simulink model "Quadrocopter_HIL_control"  (Simulink 7.4)
settings: Solver=ode45  StartTime=0.0  StopTime=7  RelTol=1e-3
values from neighbouring files (symbols this model uses):
  f1 = (I_y-I_z)/I_x    [quadrocopter_param.m]
  f2 = rot.J_z/I_x    [quadrocopter_param.m]
  f3 = (I_z-I_x)/I_y    [quadrocopter_param.m]
  f4 = rot.J_z/I_y    [quadrocopter_param.m]
  f5 = (I_x-I_y)/I_z    [quadrocopter_param.m]
  g = 9.81    [quadrocopter_param.m]
  I_x = elec.I_x+bat.I_x+2*boom.I_1x+2*boom.I_1y+2*mot.I_1x+2*mot.I_1y+                             2*rot.I_1x+2*rot.I_1y    [quadrocopter_param.m]
  I_y = elec.I_y+bat.I_y+2*boom.I_1x+2*boom.I_1y+2*mot.I_1x+2*mot.I_1y+                             2*rot.I_1x+2*rot.I_1y    [quadrocopter_param.m]
  I_z = elec.I_z+bat.I_z+4*boom.I_1z+4*mot.I_1z+4*rot.I_1z    [quadrocopter_param.m]
  m = m*1.2    [quadrocopter_param.m]
  phi0 = 0.15    [Quadrocopter_control_Driver.m]    (also in calc_stability.m = 0; control_two_angles_Driver.m; control_two_angles_and_yawrate_Driver.m; discrete_control_phi_theta_rpsi_Driver.m)
  r_phi0 = 0    [Quadrocopter_control_Driver.m]    (also in calc_stability.m; control_two_angles_Driver.m; control_two_angles_and_yawrate_Driver.m; discrete_control_phi_theta_rpsi_Driver.m)
  r_psi0 = 0    [Quadrocopter_control_Driver.m]    (also in calc_stability.m; control_two_angles_Driver.m = 0.01; control_two_angles_and_yawrate_Driver.m = 0.01; discrete_control_phi_theta_rpsi_Driver.m = 0.01)
  r_theta0 = 0    [Quadrocopter_control_Driver.m]    (also in calc_stability.m; control_two_angles_Driver.m; control_two_angles_and_yawrate_Driver.m; discrete_control_phi_theta_rpsi_Driver.m)
  theta0 = 0.15    [Quadrocopter_control_Driver.m]    (also in calc_stability.m = 0; control_two_angles_Driver.m; control_two_angles_and_yawrate_Driver.m; discrete_control_phi_theta_rpsi_Driver.m)
  Ts = 0.005    [quadrocopter_param.m]
undefined symbols (not defined in the file or in its folder): boom, Control_lib, HIL_Control
libraries: Copter_Library x6, simulink x3
settings Model: Creator=roczit00  LastModifiedBy=roczit00

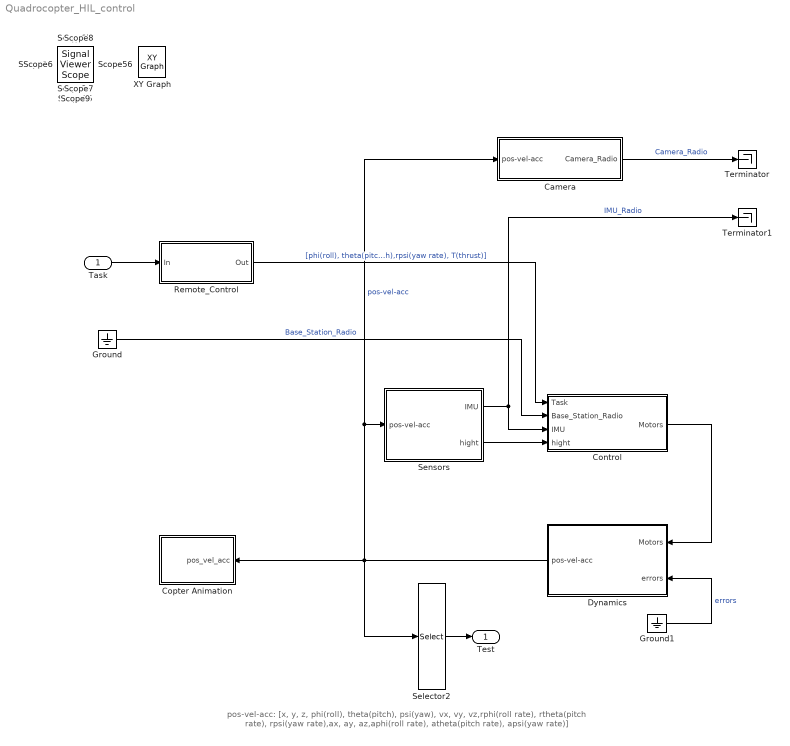
== system Quadrocopter_HIL_control ==
  note: pos-vel-acc: [x, y, z, phi(roll), theta(pitch), psi(yaw), vx, vy, vz,rphi(roll rate), rtheta(pitch rate), rpsi(yaw rate),ax, ay, az,aphi(roll rate), atheta(pitch rate), apsi(yaw rate)]
  Task : Inport  PortDimensions=4  OutDataType=fixdt(1, 16)  OutScaling=2^0
  Camera : Subsystem
  Control : Subsystem
  Copter Animation : Subsystem  mask(Quadrocopter Animation){AXES=[-100 100 -100 100 0 100], T_INT=1/25, K_VAR=Feste Position, K_POS=[5 0 1], K_ANGLE=27, A_ON=on, u_phi=on, u_theta=on, u_psi=on, u_x=off, u_y=off, u_z=off}
      mask prompts: AXES "Achsen Grenzen [xmin xmax ymin ymax zmin zmax]"; T_INT "Zeitintervall zwischen Aktualisierungen [s]:"; K_VAR "Kamera Art:"; K_POS "Ort der Kamera [xc yc zc]:"; K_ANGLE "Öffnungswinkel der Kamera [Grad]:"; A_ON "Animation Einschalten:"; u_phi "Use Input phi:"; u_theta "Use Input theta:"; u_psi "Use Input psi:"; u_x "Use Input x:"; u_y "Use Input y:"; u_z "Use Input z:"
      mask help: Erstellt eine 3-D animierte Ansicht eines Quadrocopters.
      mask init:
      | Config.axes = AXES;
      | Config.update = T_INT;
      | Config.camera_view = K_VAR;
      | Config.camera_pos = K_POS;
      | Config.view = K_ANGLE;
      | Config.Animenable = A_ON;
      | Config.phi = u_phi;
      | Config.theta = u_theta;
      | Config.psi = u_psi;
      | Config.x = u_x;
      | Config.y = u_y;
      | Config.z = u_z;
      mask Help:
      | <p>Dieser Block erstellt ein 3 dimensionales Fenster eines Quadrocopters.
      | 
      | <p><H4>Block Eingänge</H4>
      | Der Eingangsvektor bestehend aus:
      | <ul>
      | <li>X-Koordinate - Ort bezogen auf die X-Achse
      | <li>Y-Koordinate - Ort bezogen auf die Y-Achse
      | <li>Z-Koordinate - Ort bezogen auf die Z-Achse
      | <li>Psi - Yaw Drehung um die Z-Achse
      | <li>Phi - Roll Drehen um die Achse in Flugrichtung
      | <li>theta - pitch Neigung in Flugrichtung nach oben bzw. unten
      | </ul></p>
      mask StyleString: edit,edit,popup(Feste Position|Frei bewegbar),edit,edit,checkbox,checkbox,checkbox,checkbox,checkbox,checkbox,checkbox
  Dynamics : Subsystem
  Ground : Ground
  Ground1 : Ground
  Remote_Control : Subsystem
  Selector2 : Selector  InputPortWidth=19  IndexOptions=Index vector (dialog)  Indices=[4 5 6]  OutputSizes=1
  Sensors : Subsystem
  Terminator : Terminator
  Terminator1 : Terminator
  Test : Outport  OutDataType=fixdt(1, 16)  OutScaling=2^0
  Scope{,2,7..8,10,12} (6 alike) : SignalViewerScope  IOType=viewer  ZoomMode=yonly  RefreshTime=0.035000
      Scope settings: ShowLegends=on
      Scope10 settings: ShowLegends=on  SaveName=ScopeData10
      Scope12 settings: SaveName=ScopeData12
      Scope2 settings: ShowLegends=on  SaveName=ScopeData2
      Scope7 settings: SaveName=ScopeData7
      Scope8 settings: ShowLegends=on  SaveName=ScopeData8
  Scope1 : SignalViewerScope  IOType=viewer  ZoomMode=yonly  LegendLocations="1043.3333      702.66667             82      51.666667"  RefreshTime=0.035000
      settings: ShowLegends=on
  Scope11 : SignalViewerScope  IOType=viewer  ZoomMode=yonly  LegendLocations="260.3333           196            72      20.33333"  RefreshTime=0.103216
      settings: ShowLegends=on  YMin=-0.1  YMax=0.1  SaveName=ScopeData11
  Scope13 : SignalViewerScope  IOType=viewer  LegendLocations="990.2778      574.2778      159.6667      111.6667"  RefreshTime=0.035000
      settings: ShowLegends=on  SaveName=ScopeData13
  Scope14 : SignalViewerScope  IOType=viewer  ZoomMode=yonly  LegendLocations="242.3333           200            82      20.33333"  RefreshTime=0.148000
      settings: ShowLegends=on  YMin=-0.1  YMax=0.1  SaveName=ScopeData14
  Scope15 : SignalViewerScope  IOType=viewer  LegendLocations="233.3333           183            74      20.33333"  RefreshTime=0.035000
      settings: ShowLegends=on  SaveName=ScopeData15
  Scope16 : SignalViewerScope  IOType=viewer  LegendLocations="197.3333           136           106      67.33333"  RefreshTime=0.035000
      settings: ShowLegends=on  YMin=22  YMax=22  SaveName=ScopeData16
  Scope17 : SignalViewerScope  IOType=viewer  LegendLocations="180.3333           179           121      25.33333"  RefreshTime=0.035000
      settings: TickLabels=on  ShowDataMarkers=on  ShowLegends=on  TimeRange=0.01  SaveName=ScopeData17
  Scope3 : SignalViewerScope  IOType=viewer  LegendLocations="235.3333           136            72      67.33333"  RefreshTime=0.035000
      settings: ShowLegends=on  SaveName=ScopeData3
  Scope4 : SignalViewerScope  IOType=viewer  RefreshTime=0.035000
      settings: ShowLegends=on  SaveName=ScopeData4
  Scope5 : SignalViewerScope  IOType=viewer  LegendLocations="401.3333      415.6667           173      192.6667"  RefreshTime=0.035000
      settings: ShowLegends=on  SaveName=ScopeData5
  Scope6 : SignalViewerScope  IOType=viewer  RefreshTime=0.035000
      settings: ShowLegends=on  SaveName=ScopeData6
  Scope9 : SignalViewerScope  IOType=viewer  RefreshTime=0.035000
      settings: ShowLegends=on  SaveName=ScopeData9
  XY Graph : simulink/Sinks/XY Graph  IOType=viewer  SystemSampleTime=-1  xmin=-1  xmax=1  ymin=-1  ymax=1  st=-1
  wires:
  Sensors/1(IMU) -> Terminator1/1, Control/3(IMU)  "IMU_Radio"
  Sensors/2(hight) -> Control/4(hight)
  Ground1/1 -> Dynamics/2(errors)  "errors"
  Control/1(Motors) -> Dynamics/1(Motors)
  Dynamics/1(pos-vel-acc) -> Sensors/1(pos-vel-acc), Camera/1(pos-vel-acc), Selector2/1, Copter Animation/1(pos_vel_acc)  "pos-vel-acc"
  Camera/1(Camera_Radio) -> Terminator/1  "Camera_Radio"
  Ground/1 -> Control/2(Base_Station_Radio)  "Base_Station_Radio"
  Remote_Control/1(Out) -> Control/1(Task)  "[phi(roll), theta(pitch),rpsi(yaw rate), T(thrust)]"
  Selector2/1 -> Test/1
  Task/1 -> Remote_Control/1(In)

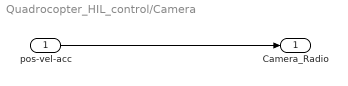
== system Quadrocopter_HIL_control/Camera ==
  pos-vel-acc : Inport  OutDataType=fixdt(1, 16)  OutScaling=2^0
  Camera_Radio : Outport  OutDataType=fixdt(1, 16)  OutScaling=2^0
  wires:
  pos-vel-acc/1 -> Camera_Radio/1

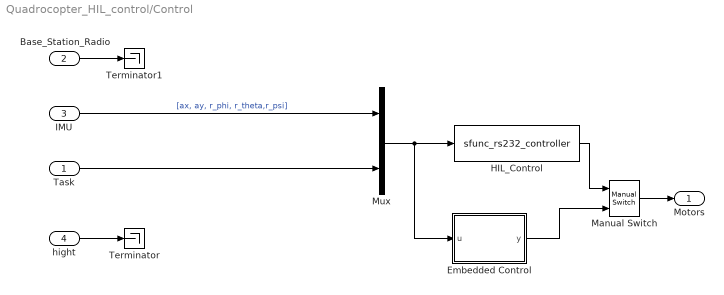
== system Quadrocopter_HIL_control/Control ==
  Task : Inport  PortDimensions=4  DataType=double  OutDataType=fixdt(1, 16)  OutScaling=2^0  OutDataTypeStr=double
  Base_Station_Radio : Inport  Port=2  OutDataType=fixdt(1, 16)  OutScaling=2^0
  IMU : Inport  Port=3  OutDataType=fixdt(1, 16)  OutScaling=2^0
  hight : Inport  Port=4  DataType=int16  OutDataType=fixdt(1, 16)  OutScaling=2^0  OutDataTypeStr=int16
  Embedded Control : Stateflow chart  AncestorBlock=Control_lib/Embedded Control
  HIL_Control : S-Function  AncestorBlock=Control_lib/HIL_Control  FunctionName=sfunc_rs232_controller  Parameters=Config  EnableBusSupport=off  mask{enabled=on}
      mask init:
      | Config.Enabled = enabled;
  Manual Switch : simulink/Signal Routing/Manual Switch  SystemSampleTime=-1  sw=1  action=0  varsize=off
  Mux : Mux  Inputs=2
  Terminator : Terminator
  Terminator1 : Terminator
  Motors : Outport  PortDimensions=4  OutDataType=fixdt(1, 16)  OutScaling=2^0
  wires:
  Base_Station_Radio/1 -> Terminator1/1
  hight/1 -> Terminator/1
  Mux/1 -> HIL_Control/1, Embedded Control/1(u)
  IMU/1 -> Mux/1  "[ax, ay, r_phi, r_theta,r_psi]"
  HIL_Control/1 -> Manual Switch/1
  Manual Switch/1 -> Motors/1
  Embedded Control/1(y) -> Manual Switch/2
  Task/1 -> Mux/2

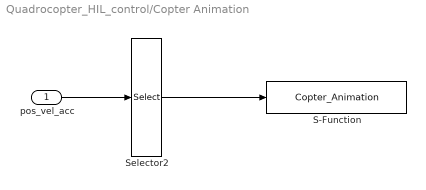
== system Quadrocopter_HIL_control/Copter Animation ==
  pos_vel_acc : Inport  PortDimensions=19  OutDataType=sfix(16)  OutScaling=2^0
  S-Function : S-Function  FunctionName=Copter_Animation  Parameters=Config  EnableBusSupport=off
  Selector2 : Selector  InputPortWidth=19  IndexOptions=Index vector (dialog)  Indices=[1 2 3 4 5 6]  OutputSizes=1
  wires:
  pos_vel_acc/1 -> Selector2/1
  Selector2/1 -> S-Function/1

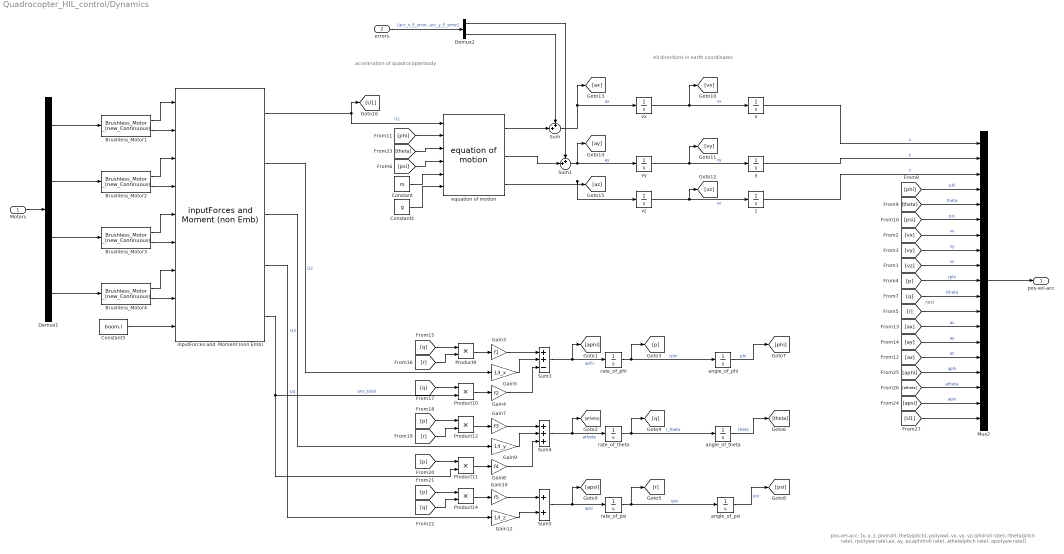
== system Quadrocopter_HIL_control/Dynamics ==
  note: rpsi
  note: pos-vel-acc: [x, y, z, phi(roll), theta(pitch), psi(yaw), vx, vy, vz,rphi(roll rate), rtheta(pitch rate), rpsi(yaw rate),ax, ay, az,aphi(roll rate), atheta(pitch rate), apsi(yaw rate)]
  note: All directions in earth coordinates
  note: acceleration of quadrocopterbody
  Motors : Inport  OutDataType=fixdt(1, 16)  OutScaling=2^0
  errors : Inport  Port=2  OutDataType=fixdt(1, 16)  OutScaling=2^0
  Brushless_Motor1 : Copter_Library/Brushless_Motor _(new_Continuous)  SystemSampleTime=-1  M_error=1
  Brushless_Motor2 : Copter_Library/Brushless_Motor _(new_Continuous)  SystemSampleTime=-1  M_error=1.03
  Brushless_Motor3 : Copter_Library/Brushless_Motor _(new_Continuous)  SystemSampleTime=-1  M_error=1
  Brushless_Motor4 : Copter_Library/Brushless_Motor _(new_Continuous)  SystemSampleTime=-1  M_error=1
  Constant : Constant  Value=m  OutDataType=fixdt(1, 16)  OutScaling=2^0
  Constant1 : Constant  Value=g  OutDataType=fixdt(1, 16)  OutScaling=2^0
  Constant3 : Constant  Value=boom.l  OutDataType=fixdt(1, 16)  OutScaling=2^0
  Demux1 : Demux
  Demux2 : Demux  Outputs=2
  Gain10 : Gain  Gain=f5  ParameterDataType=fixdt(1, 16)  ParameterScaling=2^0  OutDataType=fixdt(1, 16)  OutScaling=2^0
  Gain12 : Gain  Gain=1/I_z  ParameterDataType=fixdt(1, 16)  ParameterScaling=2^0  OutDataType=fixdt(1, 16)  OutScaling=2^0
  Gain3 : Gain  Gain=f1  ParameterDataType=fixdt(1, 16)  ParameterScaling=2^0  OutDataType=fixdt(1, 16)  OutScaling=2^0
  Gain4 : Gain  Gain=f2  ParameterDataType=fixdt(1, 16)  ParameterScaling=2^0  OutDataType=fixdt(1, 16)  OutScaling=2^0
  Gain5 : Gain  Gain=1/I_x  ParameterDataType=fixdt(1, 16)  ParameterScaling=2^0  OutDataType=fixdt(1, 16)  OutScaling=2^0
  Gain7 : Gain  Gain=f3  ParameterDataType=fixdt(1, 16)  ParameterScaling=2^0  OutDataType=fixdt(1, 16)  OutScaling=2^0
  Gain8 : Gain  Gain=f4  ParameterDataType=fixdt(1, 16)  ParameterScaling=2^0  OutDataType=fixdt(1, 16)  OutScaling=2^0
  Gain9 : Gain  Gain=1/I_y  ParameterDataType=fixdt(1, 16)  ParameterScaling=2^0  OutDataType=fixdt(1, 16)  OutScaling=2^0
  Mux2 : Mux  Inputs=19
  Product{9..12,14} (5 alike) : Product  OutDataType=fixdt(1, 16)  OutScaling=2^0  RndMeth=Zero
  Sum : Sum  Inputs=++|  OutDataType=fixdt(1, 16)  OutScaling=2^0
  Sum1 : Sum  Inputs=++|  OutDataType=fixdt(1, 16)  OutScaling=2^0
  Sum3 : Sum  Inputs=++-  OutDataType=fixdt(1, 16)  OutScaling=2^0
  Sum4 : Sum  Inputs=+++  OutDataType=fixdt(1, 16)  OutScaling=2^0
  Sum5 : Sum  OutDataType=fixdt(1, 16)  OutScaling=2^0
  angle_of_phi : Integrator  InitialCondition=phi0
  angle_of_psi : Integrator
  angle_of_theta : Integrator  InitialCondition=theta0
  equation of motion : Copter_Library/equation of motion  SystemSampleTime=-1
  inputForces and  Moment (non Emb) : Copter_Library/inputForces and  Moment (non Emb)  SystemSampleTime=-1
  rate_of_phi : Integrator  InitialCondition=r_phi0
  rate_of_psi : Integrator  InitialCondition=r_psi0
  rate_of_theta : Integrator  InitialCondition=r_theta0
  vx : Integrator
  vy : Integrator
  vz : Integrator
  x : Integrator
  y : Integrator
  z : Integrator
  pos-vel-acc : Outport  OutDataType=fixdt(1, 16)  OutScaling=2^0
  wires:
  [apsi] -> Mux2/18  "apsi"
  [atheta] -> Mux2/17  "atheta"
  [aphi] -> Mux2/16  "aphi"
  [az] -> Mux2/15  "az"
  [ay] -> Mux2/14  "ay"
  [ax] -> Mux2/13  "ax"
  [r] -> Mux2/12
  [q] -> Mux2/11  "rtheta"
  [p] -> Mux2/10  "rphi"
  [vz] -> Mux2/9  "vz"
  [vy] -> Mux2/8  "vy"
  [vx] -> Mux2/7  "vx"
  [psi] -> Mux2/6  "psi"
  [theta] -> Mux2/5  "theta"
  [phi] -> Mux2/4  "phi"
  z/1 -> Mux2/3  "z"
  Mux2/1 -> pos-vel-acc/1
  errors/1 -> Demux2/1  "[acc_x_E_error, acc_y_E_error]"
  Motors/1 -> Demux1/1
  Demux1/3 -> Brushless_Motor3/1
  Demux1/4 -> Brushless_Motor4/1
  Demux1/2 -> Brushless_Motor2/1
  Demux1/1 -> Brushless_Motor1/1
  vx/1 -> [vx], x/1  "vx"
  vy/1 -> [vy], y/1  "vy"
  vz/1 -> [vz], z/1  "vz"
  Constant3/1 -> inputForces and  Moment (non Emb)/9
  Sum5/1 -> [apsi], rate_of_psi/1  "apsi"
  inputForces and  Moment (non Emb)/4 -> Gain12/1  "U4"
  Gain12/1 -> Sum5/2
  Gain10/1 -> Sum5/1
  Product14/1 -> Gain10/1
  [q] -> Product14/2
  [p] -> Product14/1
  Sum4/1 -> [atheta], rate_of_theta/1  "atheta"
  inputForces and  Moment (non Emb)/3 -> Gain9/1  "U3"
  Gain8/1 -> Sum4/3
  Gain9/1 -> Sum4/2
  Product11/1 -> Gain8/1
  [p] -> Product11/1
  Gain7/1 -> Sum4/1
  Product12/1 -> Gain7/1
  [r] -> Product12/2
  [p] -> Product12/1
  Sum3/1 -> [aphi], rate_of_phi/1  "aphi"
  Gain4/1 -> Sum3/3
  Gain5/1 -> Sum3/2
  inputForces and  Moment (non Emb)/2 -> Gain5/1  "U2"
  Product10/1 -> Gain4/1
  [q] -> Product10/1
  Gain3/1 -> Sum3/1
  Product9/1 -> Gain3/1
  [r] -> Product9/2
  [q] -> Product9/1
  inputForces and  Moment (non Emb)/5 -> Product11/2, Product10/2  "anv_total"
  angle_of_phi/1 -> [phi]  "phi"
  angle_of_theta/1 -> [theta]  "theta"
  angle_of_psi/1 -> [psi]  "psi"
  rate_of_phi/1 -> [p], angle_of_phi/1  "rphi"
  rate_of_theta/1 -> angle_of_theta/1, [q]  "r_theta"
  rate_of_psi/1 -> angle_of_psi/1, [r]  "rpsi"
  Brushless_Motor1/1 -> inputForces and  Moment (non Emb)/1
  Brushless_Motor1/2 -> inputForces and  Moment (non Emb)/2
  Brushless_Motor2/1 -> inputForces and  Moment (non Emb)/3
  Brushless_Motor2/2 -> inputForces and  Moment (non Emb)/4
  Brushless_Motor3/1 -> inputForces and  Moment (non Emb)/5
  Brushless_Motor3/2 -> inputForces and  Moment (non Emb)/6
  Brushless_Motor4/1 -> inputForces and  Moment (non Emb)/7
  Brushless_Motor4/2 -> inputForces and  Moment (non Emb)/8
  x/1 -> Mux2/1  "x"
  y/1 -> Mux2/2  "y"
  Sum1/1 -> [ay], vy/1  "ay"
  Sum/1 -> [ax], vx/1  "ax"
  Demux2/2 -> Sum/1
  Demux2/1 -> Sum1/1
  equation of motion/3 -> [az], vz/1
  equation of motion/2 -> Sum1/2
  equation of motion/1 -> Sum/2
  inputForces and  Moment (non Emb)/1 -> equation of motion/1, [U1]  "U1"
  [phi] -> equation of motion/2
  [theta] -> equation of motion/3
  [psi] -> equation of motion/4
  Constant/1 -> equation of motion/5
  Constant1/1 -> equation of motion/6
  [U1] -> Mux2/19

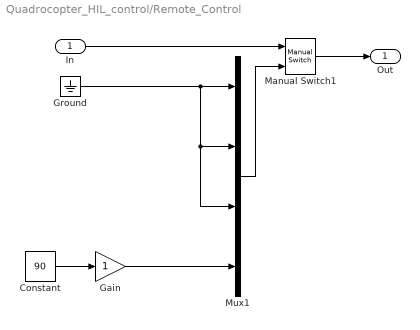
== system Quadrocopter_HIL_control/Remote_Control ==
  In : Inport  OutDataType=fixdt(1, 16)  OutScaling=2^0
  Constant : Constant  Value=90  OutDataType=fixdt(1, 16)  OutScaling=2^0
  Gain : Gain  ParameterDataType=fixdt(1, 16)  ParameterScaling=2^0  OutDataType=fixdt(1, 16)  OutScaling=2^0
  Ground : Ground
  Manual Switch1 : simulink/Signal Routing/Manual Switch  SystemSampleTime=-1  sw=0  action=0  varsize=off
  Mux1 : Mux
  Out : Outport  OutDataType=fixdt(1, 16)  OutScaling=2^0
  wires:
  In/1 -> Manual Switch1/1
  Mux1/1 -> Manual Switch1/2
  Ground/1 -> Mux1/1, Mux1/2, Mux1/3
  Manual Switch1/1 -> Out/1
  Gain/1 -> Mux1/4
  Constant/1 -> Gain/1

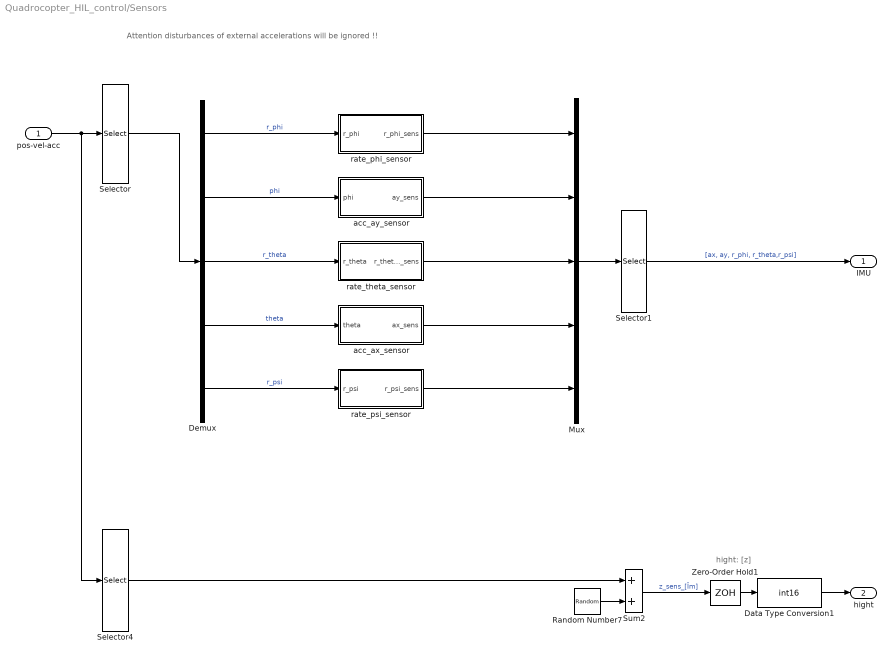
== system Quadrocopter_HIL_control/Sensors ==
  note: hight: [z]
  note: Attention disturbances of external accelerations will be ignored !!
  pos-vel-acc : Inport  PortDimensions=19  OutDataType=fixdt(1, 16)  OutScaling=2^0
  Data Type Conversion1 : DataTypeConversion  OutDataTypeMode=int16  OutDataType=fixdt(1, 16)  OutScaling=2^0  OutDataTypeStr=int16  RndMeth=Round
  Demux : Demux  Outputs=5
  Mux : Mux  Inputs=5
  Random Number7 : RandomNumber  Variance=0  SampleTime=Ts
  Selector : Selector  InputPortWidth=19  IndexOptions=Index vector (dialog)  Indices=[10 4 11 5 12]  OutputSizes=1
  Selector1 : Selector  InputPortWidth=5  IndexOptions=Index vector (dialog)  Indices=[4 2 1 3 5]  OutputSizes=1
  Selector4 : Selector  InputPortWidth=19  IndexOptions=Index vector (dialog)  Indices=[3]  OutputSizes=1
  Sum2 : Sum  OutDataType=fixdt(1, 16)  OutScaling=2^0
  Zero-Order Hold1 : ZeroOrderHold  SampleTime=Ts
  acc_ax_sensor : Subsystem
  acc_ay_sensor : Subsystem
  rate_phi_sensor : Subsystem
  rate_psi_sensor : Subsystem
  rate_theta_sensor : Subsystem
  IMU : Outport  OutDataType=fixdt(1, 16)  OutScaling=2^0
  hight : Outport  Port=2  OutDataType=fixdt(1, 16)  OutScaling=2^0
  wires:
  Random Number7/1 -> Sum2/2
  pos-vel-acc/1 -> Selector/1, Selector4/1
  Selector/1 -> Demux/1
  Selector4/1 -> Sum2/1
  Sum2/1 -> Zero-Order Hold1/1  "z_sens_[Ïm]"
  Zero-Order Hold1/1 -> Data Type Conversion1/1
  Data Type Conversion1/1 -> hight/1
  rate_phi_sensor/1(r_phi_sens) -> Mux/1
  acc_ay_sensor/1(ay_sens) -> Mux/2
  rate_theta_sensor/1(r_theta_sens) -> Mux/3
  acc_ax_sensor/1(ax_sens) -> Mux/4
  rate_psi_sensor/1(r_psi_sens) -> Mux/5
  Demux/1 -> rate_phi_sensor/1(r_phi)  "r_phi"
  Demux/2 -> acc_ay_sensor/1(phi)  "phi"
  Demux/3 -> rate_theta_sensor/1(r_theta)  "r_theta"
  Demux/4 -> acc_ax_sensor/1(theta)  "theta"
  Demux/5 -> rate_psi_sensor/1(r_psi)  "r_psi"
  Mux/1 -> Selector1/1
  Selector1/1 -> IMU/1  "[ax, ay, r_phi, r_theta,r_psi]"

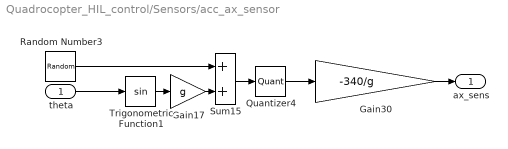
== system Quadrocopter_HIL_control/Sensors/acc_ax_sensor ==
  theta : Inport  OutDataType=fixdt(1, 16)  OutScaling=2^0
  Gain17 : Gain  Gain=g  ParameterDataType=fixdt(1, 16)  ParameterScaling=2^0  OutDataType=fixdt(1, 16)  OutScaling=2^0
  Gain30 : Gain  Gain=-340/g  ParameterDataType=fixdt(1, 16)  ParameterScaling=2^0  OutDataType=fixdt(1, 16)  OutScaling=2^0
  Quantizer4 : Quantizer  QuantizationInterval=g/340  SampleTime=Ts
  Random Number3 : RandomNumber  Variance=0.0003  Seed=676  SampleTime=Ts
  Sum15 : Sum  OutDataType=fixdt(1, 16)  OutScaling=2^0
  Trigonometric Function1 : Trigonometry
  ax_sens : Outport  OutDataType=fixdt(1, 16)  OutScaling=2^0
  wires:
  Random Number3/1 -> Sum15/1
  Sum15/1 -> Quantizer4/1
  Trigonometric Function1/1 -> Gain17/1
  Gain17/1 -> Sum15/2
  Quantizer4/1 -> Gain30/1
  theta/1 -> Trigonometric Function1/1
  Gain30/1 -> ax_sens/1

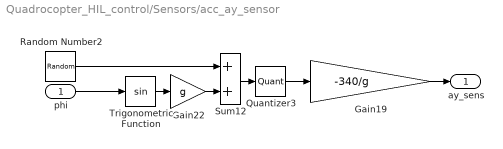
== system Quadrocopter_HIL_control/Sensors/acc_ay_sensor ==
  phi : Inport  OutDataType=fixdt(1, 16)  OutScaling=2^0
  Gain19 : Gain  Gain=-340/g  ParameterDataType=fixdt(1, 16)  ParameterScaling=2^0  OutDataType=fixdt(1, 16)  OutScaling=2^0
  Gain22 : Gain  Gain=g  ParameterDataType=fixdt(1, 16)  ParameterScaling=2^0  OutDataType=fixdt(1, 16)  OutScaling=2^0
  Quantizer3 : Quantizer  QuantizationInterval=g/340  SampleTime=Ts
  Random Number2 : RandomNumber  Variance=0.0003  Seed=4564  SampleTime=0.01
  Sum12 : Sum  OutDataType=fixdt(1, 16)  OutScaling=2^0
  Trigonometric Function : Trigonometry
  ay_sens : Outport  OutDataType=fixdt(1, 16)  OutScaling=2^0
  wires:
  Random Number2/1 -> Sum12/1
  Sum12/1 -> Quantizer3/1
  Trigonometric Function/1 -> Gain22/1
  Gain22/1 -> Sum12/2
  Quantizer3/1 -> Gain19/1
  phi/1 -> Trigonometric Function/1
  Gain19/1 -> ay_sens/1

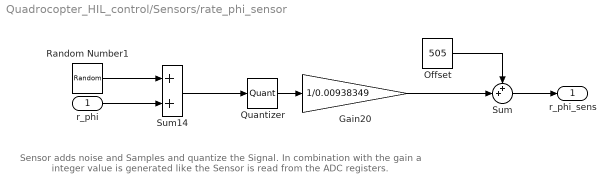
== system Quadrocopter_HIL_control/Sensors/rate_phi_sensor ==
  note: Sensor adds noise and Samples and quantize the Signal. In combination with the gain a integer value is generated
      | like the Sensor is read from the ADC registers.
  r_phi : Inport  OutDataType=fixdt(1, 16)  OutScaling=2^0
  Gain20 : Gain  Gain=1/0.00938349  ParameterDataType=fixdt(1, 16)  ParameterScaling=2^0  OutDataType=fixdt(1, 16)  OutScaling=2^0
  Offset : Constant  Value=505  OutDataType=fixdt(1, 16)  OutScaling=2^0
  Quantizer : Quantizer  QuantizationInterval=0.00938349  SampleTime=Ts
  Random Number1 : RandomNumber  Variance=3.0462e-8  Seed=45632  SampleTime=0.01
  Sum : Sum  Inputs=++|  OutDataType=fixdt(1, 16)  OutScaling=2^0
  Sum14 : Sum  OutDataType=fixdt(1, 16)  OutScaling=2^0
  r_phi_sens : Outport  OutDataType=fixdt(1, 16)  OutScaling=2^0
  wires:
  Random Number1/1 -> Sum14/1
  Sum14/1 -> Quantizer/1
  Quantizer/1 -> Gain20/1
  r_phi/1 -> Sum14/2
  Gain20/1 -> Sum/2
  Offset/1 -> Sum/1
  Sum/1 -> r_phi_sens/1

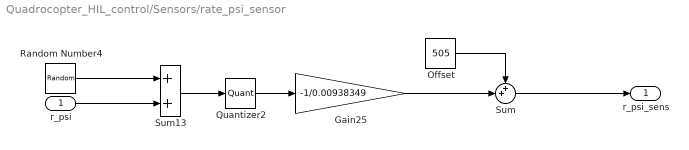
== system Quadrocopter_HIL_control/Sensors/rate_psi_sensor ==
  r_psi : Inport  OutDataType=fixdt(1, 16)  OutScaling=2^0
  Gain25 : Gain  Gain=-1/0.00938349  ParameterDataType=fixdt(1, 16)  ParameterScaling=2^0  OutDataType=fixdt(1, 16)  OutScaling=2^0
  Offset : Constant  Value=505  OutDataType=fixdt(1, 16)  OutScaling=2^0
  Quantizer2 : Quantizer  QuantizationInterval=0.00938349  SampleTime=Ts
  Random Number4 : RandomNumber  Variance=3.0462e-8  Seed=1634  SampleTime=0.01
  Sum : Sum  Inputs=++|  OutDataType=fixdt(1, 16)  OutScaling=2^0
  Sum13 : Sum  OutDataType=fixdt(1, 16)  OutScaling=2^0
  r_psi_sens : Outport  OutDataType=fixdt(1, 16)  OutScaling=2^0
  wires:
  Random Number4/1 -> Sum13/1
  Sum13/1 -> Quantizer2/1
  Quantizer2/1 -> Gain25/1
  r_psi/1 -> Sum13/2
  Offset/1 -> Sum/1
  Gain25/1 -> Sum/2
  Sum/1 -> r_psi_sens/1

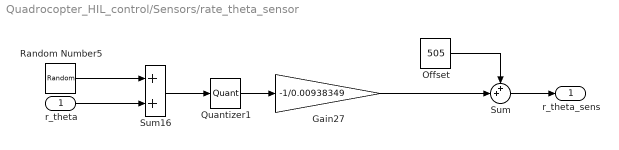
== system Quadrocopter_HIL_control/Sensors/rate_theta_sensor ==
  r_theta : Inport  OutDataType=fixdt(1, 16)  OutScaling=2^0
  Gain27 : Gain  Gain=-1/0.00938349  ParameterDataType=fixdt(1, 16)  ParameterScaling=2^0  OutDataType=fixdt(1, 16)  OutScaling=2^0
  Offset : Constant  Value=505  OutDataType=fixdt(1, 16)  OutScaling=2^0
  Quantizer1 : Quantizer  QuantizationInterval=0.00938349  SampleTime=Ts
  Random Number5 : RandomNumber  Variance=3.0462e-8  Seed=4731  SampleTime=0.01
  Sum : Sum  Inputs=++|  OutDataType=fixdt(1, 16)  OutScaling=2^0
  Sum16 : Sum  OutDataType=fixdt(1, 16)  OutScaling=2^0
  r_theta_sens : Outport  OutDataType=fixdt(1, 16)  OutScaling=2^0
  wires:
  Random Number5/1 -> Sum16/1
  Sum16/1 -> Quantizer1/1
  Quantizer1/1 -> Gain27/1
  r_theta/1 -> Sum16/2
  Offset/1 -> Sum/1
  Gain27/1 -> Sum/2
  Sum/1 -> r_theta_sens/1

== matlab function Control/Embedded Control ==
  data: u input double; y output double
function y = fcn(u)
%#eml
persistent phi_filt theta_filt M1 M2 M3 M4
%  first time initialization
if isempty(M1) 
    M1=int8(0);
end
if isempty(M2) 
    M2=int8(0);
end
if isempty(M3) 
    M3=int8(0);
end
if isempty(M4) 
    M4=int8(0);
end
if isempty(phi_filt) 
    phi_filt=0.15;
end
if isempty(theta_filt) 
    theta_filt=0.15;
end
Ts = 0.01;
Gyro_offset = 505;
% copy inputs to variables with easy to know names
Gyro_phi =  u(3)-Gyro_offset;
acc_ay = u(2);
Gyro_theta = u(4)-Gyro_offset;
acc_ax = u(1);
Gyro_psi = u(5)-Gyro_offset;
thrust = u(9);
theta_set = u(7);
phi_set = u(6);
r_psi_set = u(8);

% Set outputs to Values calculated last sample time
y = double([M1;M2;M3;M4]);

% Convert setpoint values to angles and rates
%(int16)(maxPitchAngle*(int32)(copterState->remotePitchRaw-128)/maxRemotePitch);
% Filter berechnen - ! deaktivated
phi_filt = acc_ay * 0.028852941 / 9.81; %phi_filt +Ts*((Gyro_phi * 0.00938349) + (acc_ay * 0.028852941 / 9.81 - phi_filt)*10);
theta_filt = acc_ax * 0.028852941 / 9.81;%theta_filt +Ts*((Gyro_theta * 0.00938349) + (acc_ax * 0.028852941 / 9.81 - theta_filt)*10);
% e-phi
e_phi=-(Gyro_phi * 0.00938349)*41.0+(phi_set-phi_filt)*34.9;
e_theta=-(Gyro_theta * 0.00938349)*41.0+(theta_set-theta_filt)*34.9;
e_psi=-((Gyro_psi * 0.00938349)-r_psi_set)*4.10;

%neu Ausgabewerte berechnen
M1=int8(thrust-e_theta+e_psi);
M2=int8(thrust+e_phi-e_psi);
M3=int8(thrust+e_theta+e_psi);
M4=int8(thrust-e_phi-e_psi);
